simulink model "Tank_Plant_Model"  (R2025b)
settings: Solver=FixedStepAuto  StartTime=0.0  StopTime=Sim_Duration  FixedStep=1/500  RelTol=1e-3
values from neighbouring files (symbols this model uses):
  A_3 = 13.27e-6    (= 1.327e-05)    [EReg_N2O_Simulink_Init.m]    (also in EReg_Tank_Drain_Init.m = 6e-05)
  Cd_3 = 0.6    [EReg_N2O_Simulink_Init.m]    (also in EReg_Tank_Drain_Init.m = 0.7)
  gamma_N2 = 1.4    [EReg_N2O_Simulink_Init.m]    (also in EReg_Tank_Drain_Init.m; EReg_Tank_Drain_N2O_Sim.m; N2O_Tank_Plant.m)
  K_v_4 = 0.5    [EReg_Tank_Drain_Init.m]
  m_1_0 = rho_1_0 * V_1    (= 2.35097796073)    [EReg_N2O_Simulink_Init.m]    (also in EReg_Tank_Drain_Init.m = 2.2972972973; EReg_Tank_Drain_N2O_Sim.m = params.m_1_0)
  m_2_0 = m_N2_ull_0    [EReg_N2O_Simulink_Init.m]    (also in EReg_Tank_Drain_Init.m = 0.281531531532)
  m_3_0 = m_N2O_liq_0    (= 12)    [EReg_N2O_Simulink_Init.m]    (also in EReg_Tank_Drain_Init.m = 20)
  Pst = 101325    [EReg_N2O_Simulink_Init.m]    (also in EReg_Tank_Drain_Init.m)
  R_N2 = 296    [EReg_N2O_Simulink_Init.m]    (also in EReg_Tank_Drain_Init.m; EReg_Tank_Drain_N2O_Sim.m = params.R_N2)
  rho_1_0 = P_1_0 / (R_N2 * T_0_N2)    (= 345.732053049)    [EReg_N2O_Simulink_Init.m]    (also in EReg_Tank_Drain_Init.m = 337.837837838; EReg_Tank_Drain_N2O_Sim.m = m_1_0 / V_1)
  rho_L = rhoL_init    [EReg_N2O_Simulink_Init.m]    (also in EReg_Tank_Drain_Init.m = 1000; EReg_Tank_Drain_N2O_Sim.m = T_to_rhoL(T); EregPlot.m = 1000; N2O_Tank_Plant.m = interp1_lut(T_sat_LUT, rhoL_LUT, T_N2O))
  rhost = Pst / (R_N2 * Tst)    (= 1.25320955222)    [EReg_N2O_Simulink_Init.m]    (also in EReg_Tank_Drain_Init.m)
  T_0_N2 = 293.15    [EReg_N2O_Simulink_Init.m]    (also in EReg_Tank_Drain_Init.m = 300)
  Tst = 273.15    [EReg_N2O_Simulink_Init.m]    (also in EReg_Tank_Drain_Init.m)
  V_1 = 6.8e-3    (= 0.0068)    [EReg_N2O_Simulink_Init.m]    (also in EReg_Tank_Drain_Init.m; EReg_Tank_Drain_N2O_Sim.m = params.V_1)
  V_2 = 30e-3    (= 0.03)    [EReg_N2O_Simulink_Init.m]    (also in EReg_Tank_Drain_Init.m = 0.025; EReg_Tank_Drain_N2O_Sim.m = params.V_2)
settings Model: Creator=marti  LastModifiedBy=anzashoaib
settings DataIOCC: SaveOutput=off  SaveTime=off
settings OptimizationCC: ReuseModelBlockBuffer=off
settings ModelReferenceCC: ModelReferenceMinAlgLoopOccurrences=on
settings RTWCC: GPUComputeCapability=3.5
settings GRTTargetCC: CombineOutputUpdateFcns=off

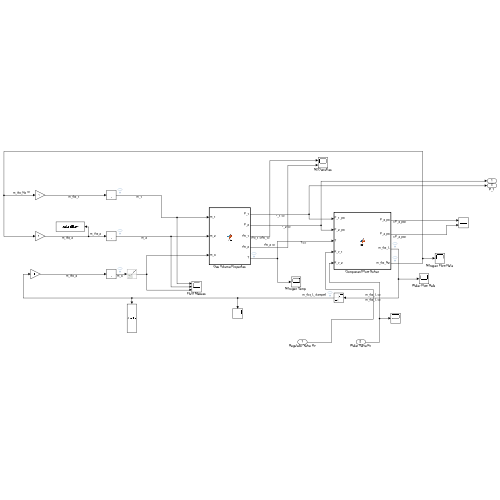
[thumbnail: Simulink's stored preview of the top-level diagram]
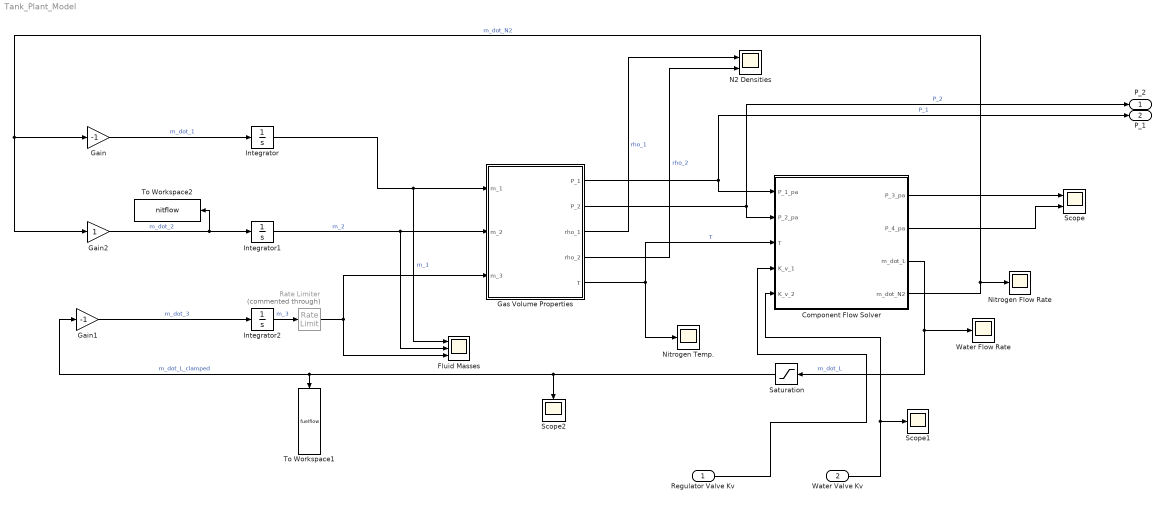
== system Tank_Plant_Model ==
  Regulator Valve Kv : Inport  OutDataTypeStr=double  PortDimensions=1  SampleTime=0
  Water Valve Kv : Inport  Port=2  OutDataTypeStr=double  PortDimensions=1  SampleTime=0
  Component Flow Solver : MATLAB Function  TreatAsAtomicUnit=on
  Fluid Masses : Scope  NumInputPorts=3
      settings: ActiveDisplayYMinimum=-0.63894  ActiveDisplayYMaximum=8.95988  DataLoggingVariableName=ScopeData4
  Gain : Gain  Gain=-1
  Gain1 : Gain  Gain=-1
  Gain2 : Gain
  Gas Volume Properties : MATLAB Function  TreatAsAtomicUnit=on
  Integrator : Integrator  InitialCondition=m_1_0
  Integrator1 : Integrator  InitialCondition=m_2_0
  Integrator2 : Integrator  InitialCondition=m_3_0
  N2 Densities : Scope  NumInputPorts=2
      settings: ActiveDisplayYMinimum=-3.2542  ActiveDisplayYMaximum=338.19949  DataLoggingVariableName=ScopeData5
  Nitrogen Flow Rate : Scope
      settings: ActiveDisplayYMinimum=-0.0436  ActiveDisplayYMaximum=0.39242
  Nitrogen Temp. : Scope
      settings: ActiveDisplayYMinimum=261.34234  ActiveDisplayYMaximum=304.2953  DataLoggingVariableName=ScopeData3
  Rate Limiter : RateLimiter  Commented=through  RisingSlewLimit=0  FallingSlewLimit=-999999999  SampleTimeMode=inherited
  Saturation : Saturate  UpperLimit=inf  LowerLimit=0
  Scope : Scope  NumInputPorts=2
      settings: ActiveDisplayYMinimum=-1.77844825772E+6  ActiveDisplayYMaximum=1.600603055574E+7  DataLoggingVariableName=ScopeData6
  Scope1 : Scope
      settings: ActiveDisplayYMinimum=-0.125  ActiveDisplayYMaximum=1.125  DataLoggingVariableName=ScopeData7
  Scope2 : Scope
      settings: ActiveDisplayYMinimum=-0.23736  ActiveDisplayYMaximum=2.13625  DataLoggingVariableName=ScopeData2
  To Workspace1 : ToWorkspace  VariableName=fuelflow  SaveFormat=Timeseries  SampleTime=-1
  To Workspace2 : ToWorkspace  VariableName=nitflow  SaveFormat=Timeseries  SampleTime=-1
  Water Flow Rate : Scope
      settings: ActiveDisplayYMinimum=-0.17675  ActiveDisplayYMaximum=1.59071
  P_2 : Outport  OutDataTypeStr=double  PortDimensions=1  SampleTime=0
  P_1 : Outport  Port=2  OutDataTypeStr=double  PortDimensions=1  SampleTime=0
  wires:
  Gas Volume Properties/1(P_1) -> Component Flow Solver/1(P_1_pa), P_1/1  "P_1"
  Gain/1 -> Integrator/1  "m_dot_1"
  Component Flow Solver/1(P_3_pa) -> Scope/1
  Integrator1/1 -> Gas Volume Properties/2(m_2), Fluid Masses/2  "m_2"
  Integrator/1 -> Gas Volume Properties/1(m_1), Fluid Masses/1  "m_1"
  Component Flow Solver/2(P_4_pa) -> Scope/2
  Gain1/1 -> Integrator2/1  "m_dot_3"
  Component Flow Solver/4(m_dot_N2) -> Gain/1, Gain2/1, Nitrogen Flow Rate/1  "m_dot_N2"
  Gain2/1 -> Integrator1/1, To Workspace2/1  "m_dot_2"
  Integrator2/1 -> Rate Limiter/1  "m_3"
  Gas Volume Properties/2(P_2) -> Component Flow Solver/2(P_2_pa), P_2/1  "P_2"
  Component Flow Solver/3(m_dot_L) -> Water Flow Rate/1, Saturation/1  "m_dot_L"
  Gas Volume Properties/4(rho_2) -> N2 Densities/2  "rho_2"
  Gas Volume Properties/3(rho_1) -> N2 Densities/1  "rho_1"
  Gas Volume Properties/5(T) -> Component Flow Solver/3(T), Nitrogen Temp./1  "T"
  Water Valve Kv/1 -> Component Flow Solver/5(K_v_2), Scope1/1
  Regulator Valve Kv/1 -> Component Flow Solver/4(K_v_1)
  Rate Limiter/1 -> Fluid Masses/3, Gas Volume Properties/3(m_3)
  Saturation/1 -> Gain1/1, To Workspace1/1, Scope2/1  "m_dot_L_clamped"

== matlab function Tank_Plant_Model/Component Flow Solver ==
  data: P_1_pa input; P_2_pa input; P_3_pa output; T input; P_4_pa output; m_dot_L output; m_dot_N2 output; K_v_1 input; K_v_2 input; Cd_3 parameter; K_v_4 parameter; rho_L parameter; R_N2 parameter; Tst parameter; rhost parameter; A_3 parameter; Pst parameter
function [P_3_pa, P_4_pa, m_dot_L, m_dot_N2] = fcn(P_1_pa, P_2_pa, T, K_v_1, K_v_2, Cd_3, K_v_4, rho_L, R_N2, Tst, rhost, A_3, Pst)
%#codegen

% This function solves for the intermediate pressures and mass flows in a
% fluid system. It replaces a non-codegen-compatible 'fsolve' call with
% two independent 1D Newton-Raphson solvers.

% --- Solver Parameters ---
MAX_ITER = 50;  % Maximum iterations for Newton's method
TOLERANCE = 1e-7; % Convergence tolerance
h = 1e-6;       % Step size for numerical derivative
P_atm_pa = 101325;
% --- Input Conversions ---
% Convert input pressures from Pascals (pa) to bar for K_v calcs
P_1 = P_1_pa * 1e-5;
P_2 = P_2_pa * 1e-5;
% Note: P_atm_pa is passed directly to calc_m_dot_b, which expects Pascals

% --- Problem Setup ---
% Calculate Specific Gravity for liquid flow
SG = rho_L / 1000.0;

% --- 1. Solve for Liquid-Side Pressure P_3 ---
% We need to find P_3 (in bar) such that: liquid_error(P_3) = 0
% where liquid_error = calc_m_dot_a(P_3) - calc_m_dot_b(P_3)

% Define the error function for the liquid side
% All parameters are passed anonymously
liquid_error_fun = @(p3) (calc_m_dot_a(p3, P_2, K_v_2, rho_L, SG) - ...
                          calc_m_dot_b(p3, Cd_3, A_3, rho_L, P_atm_pa));

% Initial guess for P_3 (in bar)
x0_P3 = 1.0; 

% Call the Newton solver
P_3_bar = newton_solver(liquid_error_fun, x0_P3, MAX_ITER, TOLERANCE, h);

% --- 2. Solve for Gas-Side Pressure P_4 ---
% We need to find P_4 (in bar) such that: gas_error(P_4) = 0
% where gas_error = calc_m_dot_c(P_4) - calc_m_dot_d(P_4)

% Define the error function for the gas side
gas_error_fun = @(p4) (calc_m_dot_c(p4, P_1, K_v_1, rhost, T, Pst, R_N2, Tst) - ...
                       calc_m_dot_d(p4, P_2, K_v_4, rhost, T, Pst, R_N2, Tst));
                       
% Initial guess for P_4 (in bar)
x0_P4 = 1.0; 

% Call the Newton solver
P_4_bar = newton_solver(gas_error_fun, x0_P4, MAX_ITER, TOLERANCE, h);

% --- 3. Calculate Final Outputs ---
% Convert pressures back to Pascals
P_3_pa = P_3_bar * 1e5;
P_4_pa = P_4_bar * 1e5;

% Calculate the final mass flow rates using the solved pressures
m_dot_L  = calc_m_dot_a(P_3_bar, P_2, K_v_2, rho_L, SG);
m_dot_N2 = calc_m_dot_c(P_4_bar, P_1, K_v_1, rhost, T, Pst, R_N2, Tst);

end

% =========================================================================
% --- NESTED HELPER FUNCTIONS (CODEGEN-COMPATIBLE) ---
% =========================================================================

function x_root = newton_solver(fun, x0, max_iter, tol, h)
% A simple 1D Newton-Raphson solver using a numerical derivative.
% It finds x such that fun(x) = 0.
    
    x_root = x0;
    for i = 1:max_iter
        % Calculate function value at current point
        f_val = fun(x_root);
        
        % Check for convergence
        if abs(f_val) < tol
            return; % Solution found
        end
        
        % Calculate function value at a small step h away
        f_val_h = fun(x_root + h);
        
        % Calculate numerical derivative (Jacobian)
        f_deriv = (f_val_h - f_val) / h;
        
        % Check for division by zero (flat gradient)
        if abs(f_deriv) < 1e-10
            % Cannot converge, return last best guess
            return;
        end
        
        % Newton's step
        x_new = x_root - f_val / f_deriv;
        
        % Check for step convergence
        if abs(x_new - x_root) < tol
            x_root = x_new;
            return; % Solution found
        end
        
        x_root = x_new;
    end
    % If loop finishes, max iterations were reached. Return last value.
end


function m_dot_a = calc_m_dot_a(P_3, P_2, K_v_2, rho_L, SG)
% Water Control Valve (m_dot_a)
% All pressures in bar
    delta_P = P_2 - P_3;
    % Use sign(delta_P) to handle potential flow reversal safely
    Q = K_v_2 * (delta_P / SG) / sqrt(abs(delta_P / SG) + 1e-9); 
    m_dot_a = Q * rho_L * (1/3600); % Convert standard flow rate to mass flow rate
end


function m_dot_b = calc_m_dot_b(P_3_bar, Cd_3, A_3, rho_L, P_atm_pa)
% Water Orifice (m_dot_b)
% P_3_bar is in bar, P_atm_pa is in Pascals
    
    % Convert P_3 from bar to Pascals for this equation
    P_3_pa = P_3_bar * 1e5;
    delta_P_pa = P_3_pa - P_atm_pa;
    
    % This formulation from your original code correctly handles flow
    % direction using sign(delta_P) * sqrt(abs(delta_P))
    m_dot_b = Cd_3 * A_3 * 2 * rho_L * delta_P_pa / sqrt(abs(2 * rho_L * delta_P_pa) + 1e-9);
end


function m_dot_c = calc_m_dot_c(P_4, P_1, K_v_1, rhost, T, Pst, R_N2, Tst)
% Regulator Valve (m_dot_c)
% All pressures in bar
    Q_N = 0.0;
    if (P_4 >= 0.528 * P_1)
        % Non-choked flow
        arg = (P_1 - P_4) * P_4 / (rhost * T);
        Q_N = K_v_1 * 514 * arg / sqrt(abs(arg) + 1e-9);
    else
        % Choked flow
        Q_N = K_v_1 * 257 * P_1 / sqrt(abs(rhost * T) + 1e-9);
    end
    m_dot_c = Q_N * (Pst / (R_N2 * Tst)) * (1/3600); % Convert standard flow rate to mass flow rate
end


function m_dot_d = calc_m_dot_d(P_4, P_2, K_v_4, rhost, T, Pst, R_N2, Tst)
% Check Valve (m_dot_d)
% All pressures in bar
    Q_N = 0.0;
    if (P_2 >= 0.528 * P_4)
        % Non-choked flow
        arg = (P_4 - P_2) * P_2 / (rhost * T);
        Q_N = K_v_4 * 514 * arg / sqrt(abs(arg) + 1e-9);
    else
        % Choked flow
        Q_N = K_v_4 * 257 * P_4 / sqrt(abs(rhost * T) + 1e-9);
    end
    m_dot_d = Q_N * (Pst / (R_N2 * Tst)) * (1/3600); % Convert standard flow rate to mass flow rate
end

== matlab function Tank_Plant_Model/Gas Volume Properties ==
  data: P_1 output; P_2 output; m_1 input; rho_1 output; m_2 input; m_3 input; rho_2 output; T output; V_1 parameter; V_2 parameter; T_0_N2 parameter; rho_1_0 parameter; gamma_N2 parameter; R_N2 parameter; rho_L parameter
function [P_1, P_2, rho_1, rho_2, T]= fcn(m_1, m_2, m_3, V_1, V_2, T_0_N2, rho_1_0, gamma_N2, R_N2, rho_L)

rho_1 = m_1/V_1; %Find the HP tank gas density
rho_2 = m_2/(V_2 - m_3/rho_L); %Find the ullage gas density
T = T_0_N2*(rho_1/rho_1_0)^(gamma_N2 - 1); %Find the ullage gas temperature (assumiong adiabatic expansion)
P_1 = rho_1*R_N2*T; %Find the HP gas pressure
P_2 = rho_2*R_N2*T; %Find the ullage gas pressure (Tank pressure)
